simulink library "lib_rfsoc_fec"  (R2020b)
settings: Solver=VariableStepAuto  StartTime=0.0  StopTime=10.0  RelTol=1e-3
undefined symbols (not defined in the file): d, fs, generator_polynomial
libraries: commseqgen3 x84, hdlsllib x83, $bdroot x33, simulink x22, dspsigops x13
(part 3 of 4)

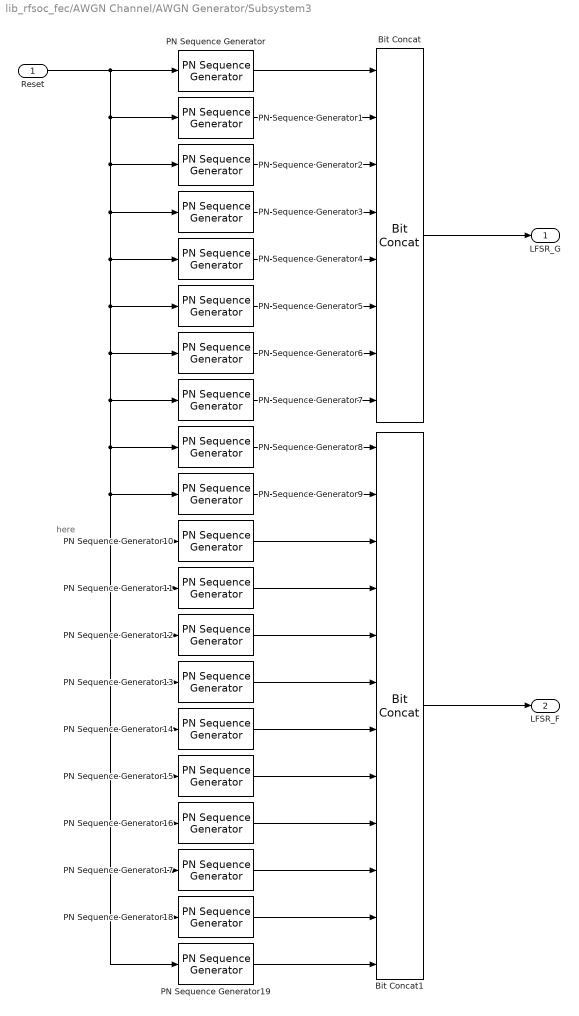
== system lib_rfsoc_fec/AWGN Channel/AWGN Generator/Subsystem3 ==
  note: here
  Reset : Inport
  Bit Concat : hdlsllib/Logic and Bit Operations/Bit Concat  numInputs=8
  Bit Concat1 : hdlsllib/Logic and Bit Operations/Bit Concat  numInputs=12
  PN Sequence Generator : commseqgen3/PN Sequence Generator  poly='z^13 + z^12 + z^11 + z^8 + 1'  ini_sta=[0 1 1 0 0 0 0 0 0 1 0 0 0]  outBitMaskSource=Dialog parameter  shift=0  outVarSiz=off  maxOutSizeMode=Dialog parameter  maxOutSize=[10 1]  Ts=-1  sampPerFrame=1  reset=on  bitPackedOutputs=off  outDataType=boolean  numPackedBits=8  bitPackDataSigned=off  bitPackedOutDType=Smallest integer
  PN Sequence Generator1 : commseqgen3/PN Sequence Generator  poly='z^13 + z^12 + z^11 + z^8 + 1'  ini_sta=[0 0 1 1 0 0 0 0 0 0 0 1 1]  outBitMaskSource=Dialog parameter  shift=0  outVarSiz=off  maxOutSizeMode=Dialog parameter  maxOutSize=[10 1]  Ts=-1  sampPerFrame=1  reset=on  bitPackedOutputs=off  outDataType=boolean  numPackedBits=8  bitPackDataSigned=off  bitPackedOutDType=Smallest integer
  PN Sequence Generator10 : commseqgen3/PN Sequence Generator  poly='z^13 + z^12 + z^11 + z^8 + 1'  ini_sta=[1 0 0 0 0 0 1 0 0 0 0 0 1]  outBitMaskSource=Dialog parameter  shift=0  outVarSiz=off  maxOutSizeMode=Dialog parameter  maxOutSize=[10 1]  Ts=-1  sampPerFrame=1  reset=on  bitPackedOutputs=off  outDataType=boolean  numPackedBits=8  bitPackDataSigned=off  bitPackedOutDType=Smallest integer
  PN Sequence Generator11 : commseqgen3/PN Sequence Generator  poly='z^13 + z^12 + z^11 + z^8 + 1'  ini_sta=[1 0 0 0 0 0 0 0 0 0 0 0 1]  outBitMaskSource=Dialog parameter  shift=0  outVarSiz=off  maxOutSizeMode=Dialog parameter  maxOutSize=[10 1]  Ts=-1  sampPerFrame=1  reset=on  bitPackedOutputs=off  outDataType=boolean  numPackedBits=8  bitPackDataSigned=off  bitPackedOutDType=Smallest integer
  PN Sequence Generator12 : commseqgen3/PN Sequence Generator  poly='z^13 + z^12 + z^11 + z^8 + 1'  ini_sta=[1 0 0 1 0 0 0 0 0 1 0 0 1]  outBitMaskSource=Dialog parameter  shift=0  outVarSiz=off  maxOutSizeMode=Dialog parameter  maxOutSize=[10 1]  Ts=-1  sampPerFrame=1  reset=on  bitPackedOutputs=off  outDataType=boolean  numPackedBits=8  bitPackDataSigned=off  bitPackedOutDType=Smallest integer
  PN Sequence Generator13 : commseqgen3/PN Sequence Generator  poly='z^13 + z^12 + z^11 + z^8 + 1'  ini_sta=[1 1 1 1 1 1 0 1 1 1 1 1 1]  outBitMaskSource=Dialog parameter  shift=0  outVarSiz=off  maxOutSizeMode=Dialog parameter  maxOutSize=[10 1]  Ts=-1  sampPerFrame=1  reset=on  bitPackedOutputs=off  outDataType=boolean  numPackedBits=8  bitPackDataSigned=off  bitPackedOutDType=Smallest integer
  PN Sequence Generator14 : commseqgen3/PN Sequence Generator  poly='z^13 + z^12 + z^11 + z^8 + 1'  ini_sta=[1 0 1 0 1 0 1 0 1 0 1 0 1]  outBitMaskSource=Dialog parameter  shift=0  outVarSiz=off  maxOutSizeMode=Dialog parameter  maxOutSize=[10 1]  Ts=-1  sampPerFrame=1  reset=on  bitPackedOutputs=off  outDataType=boolean  numPackedBits=8  bitPackDataSigned=off  bitPackedOutDType=Smallest integer
  PN Sequence Generator15 : commseqgen3/PN Sequence Generator  poly='z^13 + z^12 + z^11 + z^8 + 1'  ini_sta=[0 1 0 1 0 1 0 1 0 1 0 1 0]  outBitMaskSource=Dialog parameter  shift=0  outVarSiz=off  maxOutSizeMode=Dialog parameter  maxOutSize=[10 1]  Ts=-1  sampPerFrame=1  reset=on  bitPackedOutputs=off  outDataType=boolean  numPackedBits=8  bitPackDataSigned=off  bitPackedOutDType=Smallest integer
  PN Sequence Generator16 : commseqgen3/PN Sequence Generator  poly='z^13 + z^12 + z^11 + z^8 + 1'  ini_sta=[1 1 1 0 0 0 1 1 1 0 0 0 1]  outBitMaskSource=Dialog parameter  shift=0  outVarSiz=off  maxOutSizeMode=Dialog parameter  maxOutSize=[10 1]  Ts=-1  sampPerFrame=1  reset=on  bitPackedOutputs=off  outDataType=boolean  numPackedBits=8  bitPackDataSigned=off  bitPackedOutDType=Smallest integer
  PN Sequence Generator17 : commseqgen3/PN Sequence Generator  poly='z^13 + z^12 + z^11 + z^8 + 1'  ini_sta=[0 0 0 0 0 1 1 0 0 0 1 1 1]  outBitMaskSource=Dialog parameter  shift=0  outVarSiz=off  maxOutSizeMode=Dialog parameter  maxOutSize=[10 1]  Ts=-1  sampPerFrame=1  reset=on  bitPackedOutputs=off  outDataType=boolean  numPackedBits=8  bitPackDataSigned=off  bitPackedOutDType=Smallest integer
  PN Sequence Generator18 : commseqgen3/PN Sequence Generator  poly='z^13 + z^12 + z^11 + z^8 + 1'  ini_sta=[1 1 0 0 0 1 1 1 1 0 0 0 0]  outBitMaskSource=Dialog parameter  shift=0  outVarSiz=off  maxOutSizeMode=Dialog parameter  maxOutSize=[10 1]  Ts=-1  sampPerFrame=1  reset=on  bitPackedOutputs=off  outDataType=boolean  numPackedBits=8  bitPackDataSigned=off  bitPackedOutDType=Smallest integer
  PN Sequence Generator19 : commseqgen3/PN Sequence Generator  poly='z^13 + z^12 + z^11 + z^8 + 1'  ini_sta=[1 1 1 1 1 1 1 0 0 0 0 0 0]  outBitMaskSource=Dialog parameter  shift=0  outVarSiz=off  maxOutSizeMode=Dialog parameter  maxOutSize=[10 1]  Ts=-1  sampPerFrame=1  reset=on  bitPackedOutputs=off  outDataType=boolean  numPackedBits=8  bitPackDataSigned=off  bitPackedOutDType=Smallest integer
  PN Sequence Generator2 : commseqgen3/PN Sequence Generator  poly='z^13 + z^12 + z^11 + z^8 + 1'  ini_sta=[1 1 0 1 0 0 0 0 0 1 0 0 1]  outBitMaskSource=Dialog parameter  shift=0  outVarSiz=off  maxOutSizeMode=Dialog parameter  maxOutSize=[10 1]  Ts=-1  sampPerFrame=1  reset=on  bitPackedOutputs=off  outDataType=boolean  numPackedBits=8  bitPackDataSigned=off  bitPackedOutDType=Smallest integer
  PN Sequence Generator3 : commseqgen3/PN Sequence Generator  poly='z^13 + z^12 + z^11 + z^8 + 1'  ini_sta=[1 0 1 0 0 0 0 1 0 0 1 1 0]  outBitMaskSource=Dialog parameter  shift=0  outVarSiz=off  maxOutSizeMode=Dialog parameter  maxOutSize=[10 1]  Ts=-1  sampPerFrame=1  reset=on  bitPackedOutputs=off  outDataType=boolean  numPackedBits=8  bitPackDataSigned=off  bitPackedOutDType=Smallest integer
  PN Sequence Generator4 : commseqgen3/PN Sequence Generator  poly='z^13 + z^12 + z^11 + z^8 + 1'  ini_sta=[0 0 0 0 1 0 0 0 0 1 1 1 0]  outBitMaskSource=Dialog parameter  shift=0  outVarSiz=off  maxOutSizeMode=Dialog parameter  maxOutSize=[10 1]  Ts=-1  sampPerFrame=1  reset=on  bitPackedOutputs=off  outDataType=boolean  numPackedBits=8  bitPackDataSigned=off  bitPackedOutDType=Smallest integer
  PN Sequence Generator5 : commseqgen3/PN Sequence Generator  poly='z^13 + z^12 + z^11 + z^8 + 1'  ini_sta=[1 1 0 0 1 1 0 0 1 0 1 0 0]  outBitMaskSource=Dialog parameter  shift=0  outVarSiz=off  maxOutSizeMode=Dialog parameter  maxOutSize=[10 1]  Ts=-1  sampPerFrame=1  reset=on  bitPackedOutputs=off  outDataType=boolean  numPackedBits=8  bitPackDataSigned=off  bitPackedOutDType=Smallest integer
  PN Sequence Generator6 : commseqgen3/PN Sequence Generator  poly='z^13 + z^12 + z^11 + z^8 + 1'  ini_sta=[1 0 0 0 0 1 0 0 0 0 1 1 1]  outBitMaskSource=Dialog parameter  shift=0  outVarSiz=off  maxOutSizeMode=Dialog parameter  maxOutSize=[10 1]  Ts=-1  sampPerFrame=1  reset=on  bitPackedOutputs=off  outDataType=boolean  numPackedBits=8  bitPackDataSigned=off  bitPackedOutDType=Smallest integer
  PN Sequence Generator7 : commseqgen3/PN Sequence Generator  poly='z^13 + z^12 + z^11 + z^8 + 1'  ini_sta=[1 0 0 1 1 1 1 1 0 0 0 1 1]  outBitMaskSource=Dialog parameter  shift=0  outVarSiz=off  maxOutSizeMode=Dialog parameter  maxOutSize=[10 1]  Ts=-1  sampPerFrame=1  reset=on  bitPackedOutputs=off  outDataType=boolean  numPackedBits=8  bitPackDataSigned=off  bitPackedOutDType=Smallest integer
  PN Sequence Generator8 : commseqgen3/PN Sequence Generator  poly='z^13 + z^12 + z^11 + z^8 + 1'  ini_sta=[1 1 0 1 1 1 1 1 0 0 0 1 1]  outBitMaskSource=Dialog parameter  shift=0  outVarSiz=off  maxOutSizeMode=Dialog parameter  maxOutSize=[10 1]  Ts=-1  sampPerFrame=1  reset=on  bitPackedOutputs=off  outDataType=boolean  numPackedBits=8  bitPackDataSigned=off  bitPackedOutDType=Smallest integer
  PN Sequence Generator9 : commseqgen3/PN Sequence Generator  poly='z^13 + z^12 + z^11 + z^8 + 1'  ini_sta=[0 1 0 1 1 0 0 1 0 0 0 1 1]  outBitMaskSource=Dialog parameter  shift=0  outVarSiz=off  maxOutSizeMode=Dialog parameter  maxOutSize=[10 1]  Ts=-1  sampPerFrame=1  reset=on  bitPackedOutputs=off  outDataType=boolean  numPackedBits=8  bitPackDataSigned=off  bitPackedOutDType=Smallest integer
  LFSR_G : Outport
  LFSR_F : Outport  Port=2
  wires:
  PN Sequence Generator11/1 -> Bit Concat1/4
  PN Sequence Generator10/1 -> Bit Concat1/3
  PN Sequence Generator9/1 -> Bit Concat1/2
  PN Sequence Generator8/1 -> Bit Concat1/1
  Bit Concat1/1 -> LFSR_F/1
  Bit Concat/1 -> LFSR_G/1
  Reset/1 -> PN Sequence Generator/1, PN Sequence Generator2/1, PN Sequence Generator3/1, PN Sequence Generator8/1, PN Sequence Generator9/1, PN Sequence Generator11/1, PN Sequence Generator18/1, PN Sequence Generator19/1, PN Sequence Generator17/1, PN Sequence Generator16/1, PN Sequence Generator15/1, PN Sequence Generator14/1, PN Sequence Generator13/1, PN Sequence Generator12/1, PN Sequence Generator10/1, PN Sequence Generator7/1, PN Sequence Generator6/1, PN Sequence Generator5/1, PN Sequence Generator4/1, PN Sequence Generator1/1
  PN Sequence Generator18/1 -> Bit Concat1/11
  PN Sequence Generator13/1 -> Bit Concat1/6
  PN Sequence Generator14/1 -> Bit Concat1/7
  PN Sequence Generator12/1 -> Bit Concat1/5
  PN Sequence Generator15/1 -> Bit Concat1/8
  PN Sequence Generator16/1 -> Bit Concat1/9
  PN Sequence Generator17/1 -> Bit Concat1/10
  PN Sequence Generator19/1 -> Bit Concat1/12
  PN Sequence Generator7/1 -> Bit Concat/8
  PN Sequence Generator6/1 -> Bit Concat/7
  PN Sequence Generator5/1 -> Bit Concat/6
  PN Sequence Generator2/1 -> Bit Concat/3
  PN Sequence Generator1/1 -> Bit Concat/2
  PN Sequence Generator4/1 -> Bit Concat/5
  PN Sequence Generator3/1 -> Bit Concat/4
  PN Sequence Generator/1 -> Bit Concat/1

== system lib_rfsoc_fec/AWGN Channel/sample_and_hold/tvalid hold ==
  In1 : Inport
  Compare To Constant : simulink/Logic and Bit Operations/Compare To Constant  relop===  const=7  OutDataTypeStr=boolean
  Delay1 : Delay  DelayLength=1
  HDL Counter : hdlsllib/Sources/HDL Counter  CountType=Count limited  CountInit=0  CountStep=1  CountMax=7  CountFromType=Initial value  CountFrom=0  CountResetPort=off  CountLoadPort=off  CountEnbPort=on  CountDirPort=off  CountDataType=Unsigned  CountWordLen=3  CountFracLen=0  CountSampTime=1
  OR : Logic  Operator=OR  IconShape=distinctive  AllPortsSameDT=off  OutDataTypeStr=boolean
  Sample and Hold1 : dspsigops/Sample and Hold  trig=Rising edge  initCond=0  latchinput=off
  " " : Outport
  wires:
  HDL Counter/1 -> Compare To Constant/1
  Delay1/1 -> OR/1
  OR/1 -> Sample and Hold1/Trigger
  Compare To Constant/1 -> Delay1/1
  Sample and Hold1/1 -> " "/1, HDL Counter/1
  In1/1 -> Sample and Hold1/1, OR/2

== system lib_rfsoc_fec/QAM Mapping/Buffer/sample_and_hold ==
  s_axis_tvalid : Inport
  s_axis_tdata : Inport  Port=2
  Sample and Hold : dspsigops/Sample and Hold  trig=Rising edge  initCond=0  latchinput=off
  tvalid hold : Subsystem
  " valid_out" : Outport
  " m_axis_tdata" : Outport  Port=2
  wires:
  s_axis_tvalid/1 -> Sample and Hold/Trigger, tvalid hold/1(In1)
  tvalid hold/1(" ") -> " valid_out"/1
  s_axis_tdata/1 -> Sample and Hold/1
  Sample and Hold/1 -> " m_axis_tdata"/1

== system lib_rfsoc_fec/QAM Mapping/Buffer/sample_and_hold1 ==
  s_axis_tvalid : Inport
  s_axis_tdata : Inport  Port=2
  Sample and Hold : dspsigops/Sample and Hold  trig=Rising edge  initCond=0  latchinput=off
  tvalid hold : Subsystem
  " valid_out" : Outport
  " m_axis_tdata" : Outport  Port=2
  wires:
  Sample and Hold/1 -> " m_axis_tdata"/1
  s_axis_tdata/1 -> Sample and Hold/1
  tvalid hold/1(" ") -> " valid_out"/1
  s_axis_tvalid/1 -> tvalid hold/1(In1), Sample and Hold/Trigger

== system lib_rfsoc_fec/QAM Mapping/Buffer/sample_and_hold2 ==
  s_axis_tvalid : Inport
  s_axis_tdata : Inport  Port=2
  Sample and Hold : dspsigops/Sample and Hold  trig=Rising edge  initCond=0  latchinput=off
  tvalid hold : Subsystem
  " valid_out" : Outport
  " m_axis_tdata" : Outport  Port=2
  wires:
  s_axis_tvalid/1 -> Sample and Hold/Trigger, tvalid hold/1(In1)
  tvalid hold/1(" ") -> " valid_out"/1
  s_axis_tdata/1 -> Sample and Hold/1
  Sample and Hold/1 -> " m_axis_tdata"/1

== system lib_rfsoc_fec/QAM Mapping/Buffer/sample_and_hold3 ==
  s_axis_tvalid : Inport
  s_axis_tdata : Inport  Port=2
  Sample and Hold : dspsigops/Sample and Hold  trig=Rising edge  initCond=0  latchinput=off
  tvalid hold : Subsystem
  " valid_out" : Outport
  " m_axis_tdata" : Outport  Port=2
  wires:
  Sample and Hold/1 -> " m_axis_tdata"/1
  s_axis_tdata/1 -> Sample and Hold/1
  tvalid hold/1(" ") -> " valid_out"/1
  s_axis_tvalid/1 -> tvalid hold/1(In1), Sample and Hold/Trigger

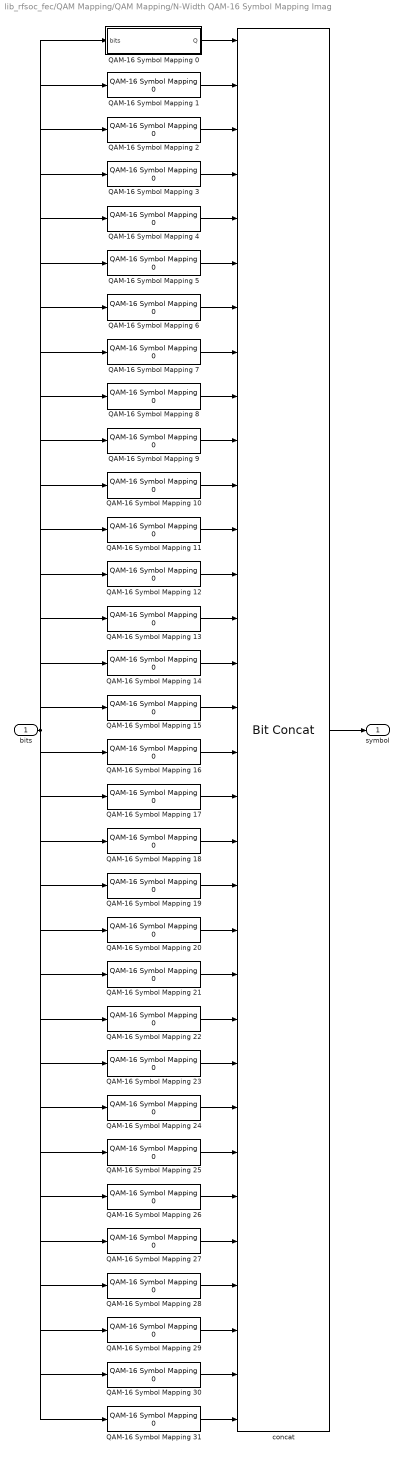
== system lib_rfsoc_fec/QAM Mapping/QAM Mapping/N-Width QAM-16 Symbol Mapping Imag ==
  bits : Inport
  QAM-16 Symbol Mapping 0 : Subsystem  mask{n=124}
  QAM-16 Symbol Mapping 1 : $bdroot/QAM Mapping/QAM Mapping/N-Width QAM-16 Symbol Mapping Imag/QAM-16 Symbol Mapping 0  n=120
  QAM-16 Symbol Mapping 10 : $bdroot/QAM Mapping/QAM Mapping/N-Width QAM-16 Symbol Mapping Imag/QAM-16 Symbol Mapping 0  n=84
  QAM-16 Symbol Mapping 11 : $bdroot/QAM Mapping/QAM Mapping/N-Width QAM-16 Symbol Mapping Imag/QAM-16 Symbol Mapping 0  n=80
  QAM-16 Symbol Mapping 12 : $bdroot/QAM Mapping/QAM Mapping/N-Width QAM-16 Symbol Mapping Imag/QAM-16 Symbol Mapping 0  n=76
  QAM-16 Symbol Mapping 13 : $bdroot/QAM Mapping/QAM Mapping/N-Width QAM-16 Symbol Mapping Imag/QAM-16 Symbol Mapping 0  n=72
  QAM-16 Symbol Mapping 14 : $bdroot/QAM Mapping/QAM Mapping/N-Width QAM-16 Symbol Mapping Imag/QAM-16 Symbol Mapping 0  n=68
  QAM-16 Symbol Mapping 15 : $bdroot/QAM Mapping/QAM Mapping/N-Width QAM-16 Symbol Mapping Imag/QAM-16 Symbol Mapping 0  n=64
  QAM-16 Symbol Mapping 16 : $bdroot/QAM Mapping/QAM Mapping/N-Width QAM-16 Symbol Mapping Imag/QAM-16 Symbol Mapping 0  n=60
  QAM-16 Symbol Mapping 17 : $bdroot/QAM Mapping/QAM Mapping/N-Width QAM-16 Symbol Mapping Imag/QAM-16 Symbol Mapping 0  n=56
  QAM-16 Symbol Mapping 18 : $bdroot/QAM Mapping/QAM Mapping/N-Width QAM-16 Symbol Mapping Imag/QAM-16 Symbol Mapping 0  n=52
  QAM-16 Symbol Mapping 19 : $bdroot/QAM Mapping/QAM Mapping/N-Width QAM-16 Symbol Mapping Imag/QAM-16 Symbol Mapping 0  n=48
  QAM-16 Symbol Mapping 2 : $bdroot/QAM Mapping/QAM Mapping/N-Width QAM-16 Symbol Mapping Imag/QAM-16 Symbol Mapping 0  n=116
  QAM-16 Symbol Mapping 20 : $bdroot/QAM Mapping/QAM Mapping/N-Width QAM-16 Symbol Mapping Imag/QAM-16 Symbol Mapping 0  n=44
  QAM-16 Symbol Mapping 21 : $bdroot/QAM Mapping/QAM Mapping/N-Width QAM-16 Symbol Mapping Imag/QAM-16 Symbol Mapping 0  n=40
  QAM-16 Symbol Mapping 22 : $bdroot/QAM Mapping/QAM Mapping/N-Width QAM-16 Symbol Mapping Imag/QAM-16 Symbol Mapping 0  n=36
  QAM-16 Symbol Mapping 23 : $bdroot/QAM Mapping/QAM Mapping/N-Width QAM-16 Symbol Mapping Imag/QAM-16 Symbol Mapping 0  n=32
  QAM-16 Symbol Mapping 24 : $bdroot/QAM Mapping/QAM Mapping/N-Width QAM-16 Symbol Mapping Imag/QAM-16 Symbol Mapping 0  n=28
  QAM-16 Symbol Mapping 25 : $bdroot/QAM Mapping/QAM Mapping/N-Width QAM-16 Symbol Mapping Imag/QAM-16 Symbol Mapping 0  n=24
  QAM-16 Symbol Mapping 26 : $bdroot/QAM Mapping/QAM Mapping/N-Width QAM-16 Symbol Mapping Imag/QAM-16 Symbol Mapping 0  n=20
  QAM-16 Symbol Mapping 27 : $bdroot/QAM Mapping/QAM Mapping/N-Width QAM-16 Symbol Mapping Imag/QAM-16 Symbol Mapping 0  n=16
  QAM-16 Symbol Mapping 28 : $bdroot/QAM Mapping/QAM Mapping/N-Width QAM-16 Symbol Mapping Imag/QAM-16 Symbol Mapping 0  n=12
  QAM-16 Symbol Mapping 29 : $bdroot/QAM Mapping/QAM Mapping/N-Width QAM-16 Symbol Mapping Imag/QAM-16 Symbol Mapping 0  n=8
  QAM-16 Symbol Mapping 3 : $bdroot/QAM Mapping/QAM Mapping/N-Width QAM-16 Symbol Mapping Imag/QAM-16 Symbol Mapping 0  n=112
  QAM-16 Symbol Mapping 30 : $bdroot/QAM Mapping/QAM Mapping/N-Width QAM-16 Symbol Mapping Imag/QAM-16 Symbol Mapping 0  n=4
  QAM-16 Symbol Mapping 31 : $bdroot/QAM Mapping/QAM Mapping/N-Width QAM-16 Symbol Mapping Imag/QAM-16 Symbol Mapping 0  n=0
  QAM-16 Symbol Mapping 4 : $bdroot/QAM Mapping/QAM Mapping/N-Width QAM-16 Symbol Mapping Imag/QAM-16 Symbol Mapping 0  n=108
  QAM-16 Symbol Mapping 5 : $bdroot/QAM Mapping/QAM Mapping/N-Width QAM-16 Symbol Mapping Imag/QAM-16 Symbol Mapping 0  n=104
  QAM-16 Symbol Mapping 6 : $bdroot/QAM Mapping/QAM Mapping/N-Width QAM-16 Symbol Mapping Imag/QAM-16 Symbol Mapping 0  n=100
  QAM-16 Symbol Mapping 7 : $bdroot/QAM Mapping/QAM Mapping/N-Width QAM-16 Symbol Mapping Imag/QAM-16 Symbol Mapping 0  n=96
  QAM-16 Symbol Mapping 8 : $bdroot/QAM Mapping/QAM Mapping/N-Width QAM-16 Symbol Mapping Imag/QAM-16 Symbol Mapping 0  n=92
  QAM-16 Symbol Mapping 9 : $bdroot/QAM Mapping/QAM Mapping/N-Width QAM-16 Symbol Mapping Imag/QAM-16 Symbol Mapping 0  n=88
  concat : hdlsllib/Logic and Bit Operations/Bit Concat  numInputs=32
  symbol : Outport
  wires:
  bits/1 -> QAM-16 Symbol Mapping 0/1(bits), QAM-16 Symbol Mapping 1/1, QAM-16 Symbol Mapping 2/1, QAM-16 Symbol Mapping 3/1, QAM-16 Symbol Mapping 4/1, QAM-16 Symbol Mapping 5/1, QAM-16 Symbol Mapping 6/1, QAM-16 Symbol Mapping 7/1, QAM-16 Symbol Mapping 8/1, QAM-16 Symbol Mapping 9/1, QAM-16 Symbol Mapping 10/1, QAM-16 Symbol Mapping 11/1, QAM-16 Symbol Mapping 12/1, QAM-16 Symbol Mapping 13/1, QAM-16 Symbol Mapping 14/1, QAM-16 Symbol Mapping 15/1, QAM-16 Symbol Mapping 16/1, QAM-16 Symbol Mapping 17/1, QAM-16 Symbol Mapping 18/1, QAM-16 Symbol Mapping 19/1, QAM-16 Symbol Mapping 20/1, QAM-16 Symbol Mapping 21/1, QAM-16 Symbol Mapping 22/1, QAM-16 Symbol Mapping 23/1, QAM-16 Symbol Mapping 24/1, QAM-16 Symbol Mapping 25/1, QAM-16 Symbol Mapping 26/1, QAM-16 Symbol Mapping 27/1, QAM-16 Symbol Mapping 28/1, QAM-16 Symbol Mapping 29/1, QAM-16 Symbol Mapping 30/1, QAM-16 Symbol Mapping 31/1
  QAM-16 Symbol Mapping 0/1(Q) -> concat/1
  QAM-16 Symbol Mapping 1/1 -> concat/2
  QAM-16 Symbol Mapping 2/1 -> concat/3
  QAM-16 Symbol Mapping 3/1 -> concat/4
  QAM-16 Symbol Mapping 4/1 -> concat/5
  QAM-16 Symbol Mapping 5/1 -> concat/6
  QAM-16 Symbol Mapping 6/1 -> concat/7
  QAM-16 Symbol Mapping 7/1 -> concat/8
  QAM-16 Symbol Mapping 8/1 -> concat/9
  QAM-16 Symbol Mapping 9/1 -> concat/10
  QAM-16 Symbol Mapping 10/1 -> concat/11
  QAM-16 Symbol Mapping 11/1 -> concat/12
  QAM-16 Symbol Mapping 12/1 -> concat/13
  QAM-16 Symbol Mapping 13/1 -> concat/14
  QAM-16 Symbol Mapping 14/1 -> concat/15
  QAM-16 Symbol Mapping 15/1 -> concat/16
  QAM-16 Symbol Mapping 16/1 -> concat/17
  QAM-16 Symbol Mapping 17/1 -> concat/18
  QAM-16 Symbol Mapping 18/1 -> concat/19
  QAM-16 Symbol Mapping 19/1 -> concat/20
  QAM-16 Symbol Mapping 20/1 -> concat/21
  QAM-16 Symbol Mapping 21/1 -> concat/22
  QAM-16 Symbol Mapping 22/1 -> concat/23
  QAM-16 Symbol Mapping 23/1 -> concat/24
  QAM-16 Symbol Mapping 24/1 -> concat/25
  QAM-16 Symbol Mapping 25/1 -> concat/26
  QAM-16 Symbol Mapping 26/1 -> concat/27
  QAM-16 Symbol Mapping 27/1 -> concat/28
  QAM-16 Symbol Mapping 28/1 -> concat/29
  QAM-16 Symbol Mapping 29/1 -> concat/30
  QAM-16 Symbol Mapping 30/1 -> concat/31
  QAM-16 Symbol Mapping 31/1 -> concat/32
  concat/1 -> symbol/1

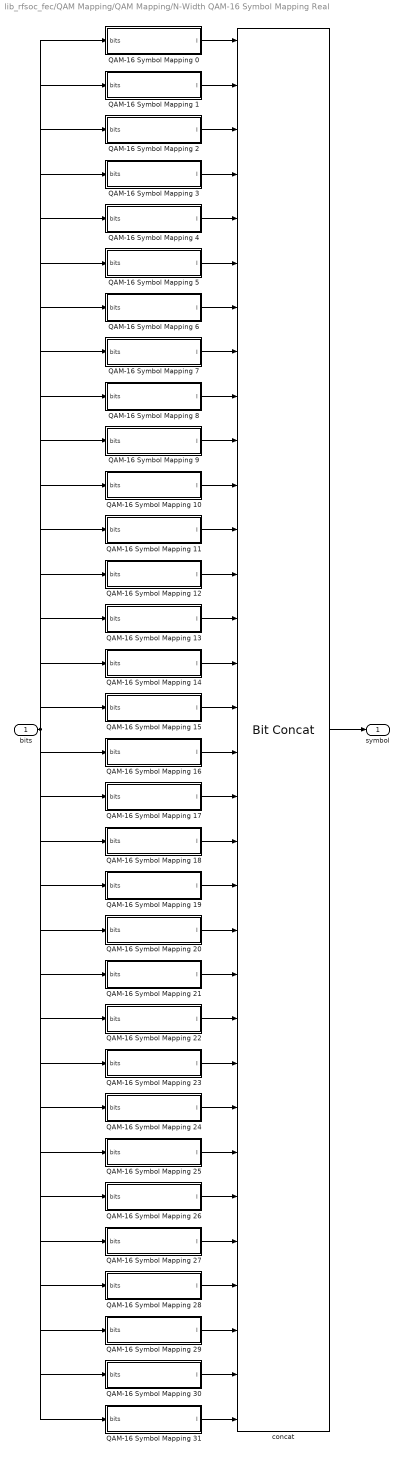
== system lib_rfsoc_fec/QAM Mapping/QAM Mapping/N-Width QAM-16 Symbol Mapping Real ==
  bits : Inport
  QAM-16 Symbol Mapping 0 : Subsystem  mask{n=124}
  QAM-16 Symbol Mapping 1 : Subsystem  mask{n=120}
  QAM-16 Symbol Mapping 10 : Subsystem  mask{n=84}
  QAM-16 Symbol Mapping 11 : Subsystem  mask{n=80}
  QAM-16 Symbol Mapping 12 : Subsystem  mask{n=76}
  QAM-16 Symbol Mapping 13 : Subsystem  mask{n=72}
  QAM-16 Symbol Mapping 14 : Subsystem  mask{n=68}
  QAM-16 Symbol Mapping 15 : Subsystem  mask{n=64}
  QAM-16 Symbol Mapping 16 : Subsystem  mask{n=60}
  QAM-16 Symbol Mapping 17 : Subsystem  mask{n=56}
  QAM-16 Symbol Mapping 18 : Subsystem  mask{n=52}
  QAM-16 Symbol Mapping 19 : Subsystem  mask{n=48}
  QAM-16 Symbol Mapping 2 : Subsystem  mask{n=116}
  QAM-16 Symbol Mapping 20 : Subsystem  mask{n=44}
  QAM-16 Symbol Mapping 21 : Subsystem  mask{n=40}
  QAM-16 Symbol Mapping 22 : Subsystem  mask{n=36}
  QAM-16 Symbol Mapping 23 : Subsystem  mask{n=32}
  QAM-16 Symbol Mapping 24 : Subsystem  mask{n=28}
  QAM-16 Symbol Mapping 25 : Subsystem  mask{n=24}
  QAM-16 Symbol Mapping 26 : Subsystem  mask{n=20}
  QAM-16 Symbol Mapping 27 : Subsystem  mask{n=16}
  QAM-16 Symbol Mapping 28 : Subsystem  mask{n=12}
  QAM-16 Symbol Mapping 29 : Subsystem  mask{n=8}
  QAM-16 Symbol Mapping 3 : Subsystem  mask{n=112}
  QAM-16 Symbol Mapping 30 : Subsystem  mask{n=4}
  QAM-16 Symbol Mapping 31 : Subsystem  mask{n=0}
  QAM-16 Symbol Mapping 4 : Subsystem  mask{n=108}
  QAM-16 Symbol Mapping 5 : Subsystem  mask{n=104}
  QAM-16 Symbol Mapping 6 : Subsystem  mask{n=100}
  QAM-16 Symbol Mapping 7 : Subsystem  mask{n=96}
  QAM-16 Symbol Mapping 8 : Subsystem  mask{n=92}
  QAM-16 Symbol Mapping 9 : Subsystem  mask{n=88}
  concat : hdlsllib/Logic and Bit Operations/Bit Concat  numInputs=32
  symbol : Outport
  wires:
  concat/1 -> symbol/1
  QAM-16 Symbol Mapping 31/1(I) -> concat/32
  QAM-16 Symbol Mapping 30/1(I) -> concat/31
  QAM-16 Symbol Mapping 29/1(I) -> concat/30
  QAM-16 Symbol Mapping 28/1(I) -> concat/29
  QAM-16 Symbol Mapping 27/1(I) -> concat/28
  QAM-16 Symbol Mapping 26/1(I) -> concat/27
  QAM-16 Symbol Mapping 25/1(I) -> concat/26
  QAM-16 Symbol Mapping 24/1(I) -> concat/25
  QAM-16 Symbol Mapping 23/1(I) -> concat/24
  QAM-16 Symbol Mapping 22/1(I) -> concat/23
  QAM-16 Symbol Mapping 21/1(I) -> concat/22
  QAM-16 Symbol Mapping 20/1(I) -> concat/21
  QAM-16 Symbol Mapping 19/1(I) -> concat/20
  QAM-16 Symbol Mapping 18/1(I) -> concat/19
  QAM-16 Symbol Mapping 17/1(I) -> concat/18
  QAM-16 Symbol Mapping 16/1(I) -> concat/17
  QAM-16 Symbol Mapping 15/1(I) -> concat/16
  QAM-16 Symbol Mapping 14/1(I) -> concat/15
  QAM-16 Symbol Mapping 13/1(I) -> concat/14
  QAM-16 Symbol Mapping 12/1(I) -> concat/13
  QAM-16 Symbol Mapping 11/1(I) -> concat/12
  QAM-16 Symbol Mapping 10/1(I) -> concat/11
  QAM-16 Symbol Mapping 9/1(I) -> concat/10
  QAM-16 Symbol Mapping 8/1(I) -> concat/9
  QAM-16 Symbol Mapping 7/1(I) -> concat/8
  QAM-16 Symbol Mapping 6/1(I) -> concat/7
  QAM-16 Symbol Mapping 5/1(I) -> concat/6
  QAM-16 Symbol Mapping 4/1(I) -> concat/5
  QAM-16 Symbol Mapping 3/1(I) -> concat/4
  QAM-16 Symbol Mapping 2/1(I) -> concat/3
  QAM-16 Symbol Mapping 1/1(I) -> concat/2
  QAM-16 Symbol Mapping 0/1(I) -> concat/1
  bits/1 -> QAM-16 Symbol Mapping 31/1(bits), QAM-16 Symbol Mapping 30/1(bits), QAM-16 Symbol Mapping 29/1(bits), QAM-16 Symbol Mapping 28/1(bits), QAM-16 Symbol Mapping 27/1(bits), QAM-16 Symbol Mapping 26/1(bits), QAM-16 Symbol Mapping 25/1(bits), QAM-16 Symbol Mapping 24/1(bits), QAM-16 Symbol Mapping 23/1(bits), QAM-16 Symbol Mapping 22/1(bits), QAM-16 Symbol Mapping 21/1(bits), QAM-16 Symbol Mapping 20/1(bits), QAM-16 Symbol Mapping 19/1(bits), QAM-16 Symbol Mapping 18/1(bits), QAM-16 Symbol Mapping 17/1(bits), QAM-16 Symbol Mapping 16/1(bits), QAM-16 Symbol Mapping 15/1(bits), QAM-16 Symbol Mapping 14/1(bits), QAM-16 Symbol Mapping 13/1(bits), QAM-16 Symbol Mapping 12/1(bits), QAM-16 Symbol Mapping 11/1(bits), QAM-16 Symbol Mapping 10/1(bits), QAM-16 Symbol Mapping 9/1(bits), QAM-16 Symbol Mapping 8/1(bits), QAM-16 Symbol Mapping 7/1(bits), QAM-16 Symbol Mapping 6/1(bits), QAM-16 Symbol Mapping 5/1(bits), QAM-16 Symbol Mapping 4/1(bits), QAM-16 Symbol Mapping 3/1(bits), QAM-16 Symbol Mapping 2/1(bits), QAM-16 Symbol Mapping 1/1(bits), QAM-16 Symbol Mapping 0/1(bits)

== system lib_rfsoc_fec/Random Number Generator/byte_count/falling_edge ==
  in : Inport
  Data Type Conversion1 : DataTypeConversion  OutDataTypeStr=boolean  SaturateOnIntegerOverflow=on  RndMeth=Zero
  Delay15 : Delay  DelayLength=1  InitialCondition=1  InputProcessing=Columns as channels (frame based)
  Logical Operator1 : Logic  Operator=NOT  Inputs=1
  Logical Operator3 : Logic
  pulse : Outport
  wires:
  Logical Operator3/1 -> pulse/1
  in/1 -> Data Type Conversion1/1
  Delay15/1 -> Logical Operator3/2
  Data Type Conversion1/1 -> Logical Operator1/1, Delay15/1
  Logical Operator1/1 -> Logical Operator3/1

== system lib_rfsoc_fec/Random Number Generator/concat/mask_generator ==
  diff : Inport
  sel : Inport  Port=2
  1-D Lookup Table{,1..3} (4 alike) : Lookup_n-D  NumberOfTableDimensions=1  BreakpointsForDimension1=[0:32]  Table=[ 0 2.^[1:32] - 1]  ExtrapMethod=Clip  InternalRulePriority=Speed  OutDataTypeStr=fixdt(0,32,0)  RndMeth=Simplest  InputSameDT=on
  Bit Concat1 : hdlsllib/Logic and Bit Operations/Bit Concat  numInputs=4
  Constant : Constant  Value=96  OutDataTypeStr=uint8  SampleTime=-1
  Constant1 : Constant  Value=2^128 - 1  OutDataTypeStr=fixdt(0,128,0)  SampleTime=-1
  Constant6 : Constant  Value=128  OutDataTypeStr=uint8  SampleTime=-1
  Constant7 : Constant  Value=64  OutDataTypeStr=uint8  SampleTime=-1
  Constant8 : Constant  Value=32  OutDataTypeStr=uint8  SampleTime=-1
  Multiport Switch : MultiPortSwitch  DataPortOrder=Zero-based contiguous  Inputs=2  zeroidx=on
  Saturation{,1..3} (4 alike) : Saturate  UpperLimit=32  LowerLimit=0
  Subtract : Sum  Inputs=+-  SaturateOnIntegerOverflow=on
  Subtract1 : Sum  Inputs=+-  SaturateOnIntegerOverflow=on
  Subtract2 : Sum  Inputs=+-  SaturateOnIntegerOverflow=on
  Subtract3 : Sum  Inputs=+-  OutDataTypeStr=uint8
  falling_edge : Subsystem
  mask : Outport
  wires:
  falling_edge/1(pulse) -> Multiport Switch/1
  sel/1 -> falling_edge/1(in)
  1-D Lookup Table1/1 -> Bit Concat1/2
  1-D Lookup Table/1 -> Bit Concat1/1
  1-D Lookup Table3/1 -> Bit Concat1/4
  Constant/1 -> Subtract/2
  Subtract/1 -> Saturation/1
  diff/1 -> Subtract3/2
  Subtract2/1 -> Saturation2/1
  Subtract1/1 -> Saturation1/1
  Constant7/1 -> Subtract1/2
  Saturation/1 -> 1-D Lookup Table/1
  1-D Lookup Table2/1 -> Bit Concat1/3
  Saturation1/1 -> 1-D Lookup Table1/1
  Saturation2/1 -> 1-D Lookup Table2/1
  Saturation3/1 -> 1-D Lookup Table3/1
  Constant8/1 -> Subtract2/2
  Bit Concat1/1 -> Multiport Switch/3
  Subtract3/1 -> Saturation3/1, Subtract2/1, Subtract1/1, Subtract/1
  Constant6/1 -> Subtract3/1
  Constant1/1 -> Multiport Switch/2
  Multiport Switch/1 -> mask/1

== system lib_rfsoc_fec/Random Number Generator/interface_creator/latch1 ==
  data_in : Inport
  en : Inport  Port=2
  Delay16 : Delay  DelayLength=1
  Multiport Switch : MultiPortSwitch  DataPortOrder=Zero-based contiguous  Inputs=2  zeroidx=on
  data_out : Outport
  wires:
  Multiport Switch/1 -> data_out/1, Delay16/1
  Delay16/1 -> Multiport Switch/2
  en/1 -> Multiport Switch/1
  data_in/1 -> Multiport Switch/3

== system lib_rfsoc_fec/Random Number Generator/interface_creator/latch10 ==
  data_in : Inport
  en : Inport  Port=2
  Delay16 : Delay  DelayLength=1
  Multiport Switch : MultiPortSwitch  DataPortOrder=Zero-based contiguous  Inputs=2  zeroidx=on
  data_out : Outport
  wires:
  en/1 -> Multiport Switch/1
  data_in/1 -> Multiport Switch/3
  Delay16/1 -> Multiport Switch/2
  Multiport Switch/1 -> Delay16/1, data_out/1

== system lib_rfsoc_fec/Random Number Generator/interface_creator/latch2 ==
  data_in : Inport
  en : Inport  Port=2
  Delay16 : Delay  DelayLength=1
  Multiport Switch : MultiPortSwitch  DataPortOrder=Zero-based contiguous  Inputs=2  zeroidx=on
  data_out : Outport
  wires:
  data_in/1 -> Multiport Switch/3
  en/1 -> Multiport Switch/1
  Delay16/1 -> Multiport Switch/2
  Multiport Switch/1 -> Delay16/1, data_out/1

== system lib_rfsoc_fec/Random Number Generator/interface_creator/latch4 ==
  data : Inport
  reset : Inport  Port=2
  Delay16 : Delay  DelayLength=1
  Multiport Switch : MultiPortSwitch  DataPortOrder=Zero-based contiguous  Inputs=2  zeroidx=on
  OR1 : Logic  Operator=OR  IconShape=distinctive  AllPortsSameDT=off  OutDataTypeStr=boolean
  data_out : Outport
  wires:
  Multiport Switch/1 -> data_out/1, Delay16/1
  Delay16/1 -> Multiport Switch/2
  OR1/1 -> Multiport Switch/1
  reset/1 -> OR1/1
  data/1 -> OR1/2, Multiport Switch/3

== system lib_rfsoc_fec/Random Number Generator/interface_creator/latch5 ==
  data : Inport
  reset : Inport  Port=2
  Delay16 : Delay  DelayLength=1
  Multiport Switch : MultiPortSwitch  DataPortOrder=Zero-based contiguous  Inputs=2  zeroidx=on
  OR1 : Logic  Operator=OR  IconShape=distinctive  AllPortsSameDT=off  OutDataTypeStr=boolean
  data_out : Outport
  wires:
  data/1 -> Multiport Switch/3, OR1/2
  reset/1 -> OR1/1
  OR1/1 -> Multiport Switch/1
  Delay16/1 -> Multiport Switch/2
  Multiport Switch/1 -> Delay16/1, data_out/1

== system lib_rfsoc_fec/Random Number Generator/interface_creator/latch6 ==
  data : Inport
  reset : Inport  Port=2
  Delay16 : Delay  DelayLength=1
  Multiport Switch : MultiPortSwitch  DataPortOrder=Zero-based contiguous  Inputs=2  zeroidx=on
  OR1 : Logic  Operator=OR  IconShape=distinctive  AllPortsSameDT=off  OutDataTypeStr=boolean
  data_out : Outport
  wires:
  Multiport Switch/1 -> data_out/1, Delay16/1
  Delay16/1 -> Multiport Switch/2
  OR1/1 -> Multiport Switch/1
  reset/1 -> OR1/1
  data/1 -> OR1/2, Multiport Switch/3

== system lib_rfsoc_fec/Random Number Generator/interface_creator/latch7 ==
  data_in : Inport
  en : Inport  Port=2
  Delay16 : Delay  DelayLength=1
  Multiport Switch : MultiPortSwitch  DataPortOrder=Zero-based contiguous  Inputs=2  zeroidx=on
  data_out : Outport
  wires:
  en/1 -> Multiport Switch/1
  Multiport Switch/1 -> data_out/1, Delay16/1
  Delay16/1 -> Multiport Switch/2
  data_in/1 -> Multiport Switch/3

== system lib_rfsoc_fec/Random Number Generator/interface_creator/latch8 ==
  data_in : Inport
  en : Inport  Port=2
  Delay16 : Delay  DelayLength=1
  Multiport Switch : MultiPortSwitch  DataPortOrder=Zero-based contiguous  Inputs=2  zeroidx=on
  data_out : Outport
  wires:
  en/1 -> Multiport Switch/1
  data_in/1 -> Multiport Switch/3
  Delay16/1 -> Multiport Switch/2
  Multiport Switch/1 -> Delay16/1, data_out/1

== system lib_rfsoc_fec/Random Number Generator/interface_creator/latch9 ==
  data_in : Inport
  en : Inport  Port=2
  Delay16 : Delay  DelayLength=1
  Multiport Switch : MultiPortSwitch  DataPortOrder=Zero-based contiguous  Inputs=2  zeroidx=on
  data_out : Outport
  wires:
  Multiport Switch/1 -> data_out/1, Delay16/1
  Delay16/1 -> Multiport Switch/2
  data_in/1 -> Multiport Switch/3
  en/1 -> Multiport Switch/1

== system lib_rfsoc_fec/Random Number Generator/interface_creator/rising_edge ==
  in : Inport
  Data Type Conversion1 : DataTypeConversion  OutDataTypeStr=boolean  SaturateOnIntegerOverflow=on  RndMeth=Zero
  Delay15 : Delay  DelayLength=1  InitialCondition=1  InputProcessing=Columns as channels (frame based)
  Logical Operator2 : Logic  Operator=NOT  Inputs=1
  Logical Operator3 : Logic
  pulse : Outport
  wires:
  Logical Operator2/1 -> Logical Operator3/2
  in/1 -> Data Type Conversion1/1
  Data Type Conversion1/1 -> Logical Operator3/1, Delay15/1
  Logical Operator3/1 -> pulse/1
  Delay15/1 -> Logical Operator2/1

== system lib_rfsoc_fec/Soft Demodulation/Soft Demodulation/Subsystem ==
  enb : Inport
  1-D Lookup Table : Lookup_n-D  NumberOfTableDimensions=1  BreakpointsForDimension1=[0:3]  IndexSearchMethod=Evenly spaced points  Table=[3 3 3 -1]  InterpMethod=Flat  DiagnosticForOutOfRangeInput=Error  InternalRulePriority=Speed  OutDataTypeStr=fixdt(1,3,0)  RndMeth=Simplest  InputSameDT=on
  1-D Lookup Table1 : Lookup_n-D  NumberOfTableDimensions=1  BreakpointsForDimension1=[0:3]  IndexSearchMethod=Evenly spaced points  Table=[1 1 3 -1]  InterpMethod=Flat  DiagnosticForOutOfRangeInput=Error  InternalRulePriority=Speed  OutDataTypeStr=fixdt(1,3,0)  RndMeth=Simplest  InputSameDT=on
  1-D Lookup Table2 : Lookup_n-D  NumberOfTableDimensions=1  BreakpointsForDimension1=[0:3]  IndexSearchMethod=Evenly spaced points  Table=[-1 -1 3 -1]  InterpMethod=Flat  DiagnosticForOutOfRangeInput=Error  InternalRulePriority=Speed  OutDataTypeStr=fixdt(1,3,0)  RndMeth=Simplest  InputSameDT=on
  1-D Lookup Table3 : Lookup_n-D  NumberOfTableDimensions=1  BreakpointsForDimension1=[0:3]  IndexSearchMethod=Evenly spaced points  Table=[-3 -3 3 -1]  InterpMethod=Flat  DiagnosticForOutOfRangeInput=Error  InternalRulePriority=Speed  OutDataTypeStr=fixdt(1,3,0)  RndMeth=Simplest  InputSameDT=on
  1-D Lookup Table4 : Lookup_n-D  NumberOfTableDimensions=1  BreakpointsForDimension1=[0:3]  IndexSearchMethod=Evenly spaced points  Table=[3 3 -3 -3]  InterpMethod=Flat  DiagnosticForOutOfRangeInput=Error  InternalRulePriority=Speed  OutDataTypeStr=fixdt(1,3,0)  RndMeth=Simplest  InputSameDT=on
  1-D Lookup Table5 : Lookup_n-D  NumberOfTableDimensions=1  BreakpointsForDimension1=[0:3]  IndexSearchMethod=Evenly spaced points  Table=[1 1 -3 -3]  InterpMethod=Flat  DiagnosticForOutOfRangeInput=Error  InternalRulePriority=Speed  OutDataTypeStr=fixdt(1,3,0)  RndMeth=Simplest  InputSameDT=on
  1-D Lookup Table6 : Lookup_n-D  NumberOfTableDimensions=1  BreakpointsForDimension1=[0:3]  IndexSearchMethod=Evenly spaced points  Table=[-1 -1 -3 -3]  InterpMethod=Flat  DiagnosticForOutOfRangeInput=Error  InternalRulePriority=Speed  OutDataTypeStr=fixdt(1,3,0)  RndMeth=Simplest  InputSameDT=on
  1-D Lookup Table7 : Lookup_n-D  NumberOfTableDimensions=1  BreakpointsForDimension1=[0:3]  IndexSearchMethod=Evenly spaced points  Table=[-3 -3 -3 -3]  InterpMethod=Flat  DiagnosticForOutOfRangeInput=Error  InternalRulePriority=Speed  OutDataTypeStr=fixdt(1,3,0)  RndMeth=Simplest  InputSameDT=on
  Out1 : Outport
  Out2 : Outport  Port=2
  Out3 : Outport  Port=3
  Out4 : Outport  Port=4
  Out5 : Outport  Port=5
  Out6 : Outport  Port=6
  Out7 : Outport  Port=7
  Out8 : Outport  Port=8
  wires:
  1-D Lookup Table7/1 -> Out8/1
  1-D Lookup Table2/1 -> Out3/1
  1-D Lookup Table/1 -> Out1/1
  1-D Lookup Table5/1 -> Out6/1
  1-D Lookup Table4/1 -> Out5/1
  1-D Lookup Table1/1 -> Out2/1
  1-D Lookup Table3/1 -> Out4/1
  enb/1 -> 1-D Lookup Table7/1, 1-D Lookup Table6/1, 1-D Lookup Table5/1, 1-D Lookup Table4/1, 1-D Lookup Table/1, 1-D Lookup Table1/1, 1-D Lookup Table2/1, 1-D Lookup Table3/1
  1-D Lookup Table6/1 -> Out7/1

== system lib_rfsoc_fec/Soft Demodulation/Soft Demodulation/Subsystem1 ==
  a : Inport
  b : Inport  Port=2
  a1 : Inport  Port=3
  b1 : Inport  Port=4
  a2 : Inport  Port=5
  b2 : Inport  Port=6
  a3 : Inport  Port=7
  b3 : Inport  Port=8
  get_min1 : Subsystem
  get_min2 : Subsystem
  get_min3 : Subsystem
  get_min4 : Subsystem
  get_min5 : Subsystem
  get_min6 : Subsystem
  get_min7 : Subsystem
  min : Outport
  wires:
  a2/1 -> get_min3/1(a)
  b/1 -> get_min1/2(b)
  a1/1 -> get_min2/1(a)
  b3/1 -> get_min4/2(b)
  get_min7/1(min) -> min/1
  get_min1/1(min) -> get_min5/1(a)
  a3/1 -> get_min4/1(a)
  get_min4/1(min) -> get_min6/2(b)
  get_min2/1(min) -> get_min5/2(b)
  b1/1 -> get_min2/2(b)
  get_min3/1(min) -> get_min6/1(a)
  get_min6/1(min) -> get_min7/2(b)
  a/1 -> get_min1/1(a)
  b2/1 -> get_min3/2(b)
  get_min5/1(min) -> get_min7/1(a)

== system lib_rfsoc_fec/Soft Demodulation/Soft Demodulation/Subsystem3 ==
  enb : Inport
  1-D Lookup Table : Lookup_n-D  NumberOfTableDimensions=1  BreakpointsForDimension1=[0:3]  IndexSearchMethod=Evenly spaced points  Table=[-3 1 3 3]  InterpMethod=Flat  DiagnosticForOutOfRangeInput=Error  InternalRulePriority=Speed  OutDataTypeStr=fixdt(1,3,0)  RndMeth=Simplest  InputSameDT=on
  1-D Lookup Table1 : Lookup_n-D  NumberOfTableDimensions=1  BreakpointsForDimension1=[0:3]  IndexSearchMethod=Evenly spaced points  Table=[-3 1 1 1]  InterpMethod=Flat  DiagnosticForOutOfRangeInput=Error  InternalRulePriority=Speed  OutDataTypeStr=fixdt(1,3,0)  RndMeth=Simplest  InputSameDT=on
  1-D Lookup Table2 : Lookup_n-D  NumberOfTableDimensions=1  BreakpointsForDimension1=[0:3]  IndexSearchMethod=Evenly spaced points  Table=[-3 1 -1 -1]  InterpMethod=Flat  DiagnosticForOutOfRangeInput=Error  InternalRulePriority=Speed  OutDataTypeStr=fixdt(1,3,0)  RndMeth=Simplest  InputSameDT=on
  1-D Lookup Table3 : Lookup_n-D  NumberOfTableDimensions=1  BreakpointsForDimension1=[0:3]  IndexSearchMethod=Evenly spaced points  Table=[-3 1 -3 -3]  InterpMethod=Flat  DiagnosticForOutOfRangeInput=Error  InternalRulePriority=Speed  OutDataTypeStr=fixdt(1,3,0)  RndMeth=Simplest  InputSameDT=on
  1-D Lookup Table4 : Lookup_n-D  NumberOfTableDimensions=1  BreakpointsForDimension1=[0:3]  IndexSearchMethod=Evenly spaced points  Table=[3 3 3 3]  InterpMethod=Flat  DiagnosticForOutOfRangeInput=Error  InternalRulePriority=Speed  OutDataTypeStr=fixdt(1,3,0)  RndMeth=Simplest  InputSameDT=on
  1-D Lookup Table5 : Lookup_n-D  NumberOfTableDimensions=1  BreakpointsForDimension1=[0:3]  IndexSearchMethod=Evenly spaced points  Table=[3 3 1 1]  InterpMethod=Flat  DiagnosticForOutOfRangeInput=Error  InternalRulePriority=Speed  OutDataTypeStr=fixdt(1,3,0)  RndMeth=Simplest  InputSameDT=on
  1-D Lookup Table6 : Lookup_n-D  NumberOfTableDimensions=1  BreakpointsForDimension1=[0:3]  IndexSearchMethod=Evenly spaced points  Table=[3 3 -1 -1]  InterpMethod=Flat  DiagnosticForOutOfRangeInput=Error  InternalRulePriority=Speed  OutDataTypeStr=fixdt(1,3,0)  RndMeth=Simplest  InputSameDT=on
  1-D Lookup Table7 : Lookup_n-D  NumberOfTableDimensions=1  BreakpointsForDimension1=[0:3]  IndexSearchMethod=Evenly spaced points  Table=[3 3 -3 -3]  InterpMethod=Flat  DiagnosticForOutOfRangeInput=Error  InternalRulePriority=Speed  OutDataTypeStr=fixdt(1,3,0)  RndMeth=Simplest  InputSameDT=on
  Out1 : Outport
  Out2 : Outport  Port=2
  Out3 : Outport  Port=3
  Out4 : Outport  Port=4
  Out5 : Outport  Port=5
  Out6 : Outport  Port=6
  Out7 : Outport  Port=7
  Out8 : Outport  Port=8
  wires:
  1-D Lookup Table7/1 -> Out8/1
  1-D Lookup Table2/1 -> Out3/1
  1-D Lookup Table/1 -> Out1/1
  1-D Lookup Table5/1 -> Out6/1
  1-D Lookup Table4/1 -> Out5/1
  1-D Lookup Table1/1 -> Out2/1
  1-D Lookup Table3/1 -> Out4/1
  enb/1 -> 1-D Lookup Table3/1, 1-D Lookup Table2/1, 1-D Lookup Table1/1, 1-D Lookup Table/1, 1-D Lookup Table7/1, 1-D Lookup Table6/1, 1-D Lookup Table5/1, 1-D Lookup Table4/1
  1-D Lookup Table6/1 -> Out7/1

== system lib_rfsoc_fec/Soft Demodulation/Soft Demodulation/Subsystem4 ==
  enb : Inport
  1-D Lookup Table : Lookup_n-D  NumberOfTableDimensions=1  BreakpointsForDimension1=[0:3]  IndexSearchMethod=Evenly spaced points  Table=[1 -3 3 3]  InterpMethod=Flat  DiagnosticForOutOfRangeInput=Error  InternalRulePriority=Speed  OutDataTypeStr=fixdt(1,3,0)  RndMeth=Simplest  InputSameDT=on
  1-D Lookup Table1 : Lookup_n-D  NumberOfTableDimensions=1  BreakpointsForDimension1=[0:3]  IndexSearchMethod=Evenly spaced points  Table=[1 -3 1 1]  InterpMethod=Flat  DiagnosticForOutOfRangeInput=Error  InternalRulePriority=Speed  OutDataTypeStr=fixdt(1,3,0)  RndMeth=Simplest  InputSameDT=on
  1-D Lookup Table2 : Lookup_n-D  NumberOfTableDimensions=1  BreakpointsForDimension1=[0:3]  IndexSearchMethod=Evenly spaced points  Table=[1 -3 -1 -1]  InterpMethod=Flat  DiagnosticForOutOfRangeInput=Error  InternalRulePriority=Speed  OutDataTypeStr=fixdt(1,3,0)  RndMeth=Simplest  InputSameDT=on
  1-D Lookup Table3 : Lookup_n-D  NumberOfTableDimensions=1  BreakpointsForDimension1=[0:3]  IndexSearchMethod=Evenly spaced points  Table=[1 -3 -3 -3]  InterpMethod=Flat  DiagnosticForOutOfRangeInput=Error  InternalRulePriority=Speed  OutDataTypeStr=fixdt(1,3,0)  RndMeth=Simplest  InputSameDT=on
  1-D Lookup Table4 : Lookup_n-D  NumberOfTableDimensions=1  BreakpointsForDimension1=[0:3]  IndexSearchMethod=Evenly spaced points  Table=[-1 -1 3 3]  InterpMethod=Flat  DiagnosticForOutOfRangeInput=Error  InternalRulePriority=Speed  OutDataTypeStr=fixdt(1,3,0)  RndMeth=Simplest  InputSameDT=on
  1-D Lookup Table5 : Lookup_n-D  NumberOfTableDimensions=1  BreakpointsForDimension1=[0:3]  IndexSearchMethod=Evenly spaced points  Table=[-1 -1 1 1]  InterpMethod=Flat  DiagnosticForOutOfRangeInput=Error  InternalRulePriority=Speed  OutDataTypeStr=fixdt(1,3,0)  RndMeth=Simplest  InputSameDT=on
  1-D Lookup Table6 : Lookup_n-D  NumberOfTableDimensions=1  BreakpointsForDimension1=[0:3]  IndexSearchMethod=Evenly spaced points  Table=[-1 -1 -1 -1]  InterpMethod=Flat  DiagnosticForOutOfRangeInput=Error  InternalRulePriority=Speed  OutDataTypeStr=fixdt(1,3,0)  RndMeth=Simplest  InputSameDT=on
  1-D Lookup Table7 : Lookup_n-D  NumberOfTableDimensions=1  BreakpointsForDimension1=[0:3]  IndexSearchMethod=Evenly spaced points  Table=[-1 -1 -3 -3]  InterpMethod=Flat  DiagnosticForOutOfRangeInput=Error  InternalRulePriority=Speed  OutDataTypeStr=fixdt(1,3,0)  RndMeth=Simplest  InputSameDT=on
  Out1 : Outport
  Out2 : Outport  Port=2
  Out3 : Outport  Port=3
  Out4 : Outport  Port=4
  Out5 : Outport  Port=5
  Out6 : Outport  Port=6
  Out7 : Outport  Port=7
  Out8 : Outport  Port=8
  wires:
  1-D Lookup Table6/1 -> Out7/1
  enb/1 -> 1-D Lookup Table/1, 1-D Lookup Table1/1, 1-D Lookup Table2/1, 1-D Lookup Table3/1, 1-D Lookup Table4/1, 1-D Lookup Table5/1, 1-D Lookup Table6/1, 1-D Lookup Table7/1
  1-D Lookup Table3/1 -> Out4/1
  1-D Lookup Table1/1 -> Out2/1
  1-D Lookup Table4/1 -> Out5/1
  1-D Lookup Table5/1 -> Out6/1
  1-D Lookup Table/1 -> Out1/1
  1-D Lookup Table2/1 -> Out3/1
  1-D Lookup Table7/1 -> Out8/1

== system lib_rfsoc_fec/Soft Demodulation/Soft Demodulation/Subsystem5 ==
  enb : Inport
  1-D Lookup Table : Lookup_n-D  NumberOfTableDimensions=1  BreakpointsForDimension1=[0:3]  IndexSearchMethod=Evenly spaced points  Table=[3 3 1 3]  InterpMethod=Flat  DiagnosticForOutOfRangeInput=Error  InternalRulePriority=Speed  OutDataTypeStr=fixdt(1,3,0)  RndMeth=Simplest  InputSameDT=on
  1-D Lookup Table1 : Lookup_n-D  NumberOfTableDimensions=1  BreakpointsForDimension1=[0:3]  IndexSearchMethod=Evenly spaced points  Table=[1 1 1 3]  InterpMethod=Flat  DiagnosticForOutOfRangeInput=Error  InternalRulePriority=Speed  OutDataTypeStr=fixdt(1,3,0)  RndMeth=Simplest  InputSameDT=on
  1-D Lookup Table2 : Lookup_n-D  NumberOfTableDimensions=1  BreakpointsForDimension1=[0:3]  IndexSearchMethod=Evenly spaced points  Table=[-1 -1 1 3]  InterpMethod=Flat  DiagnosticForOutOfRangeInput=Error  InternalRulePriority=Speed  OutDataTypeStr=fixdt(1,3,0)  RndMeth=Simplest  InputSameDT=on
  1-D Lookup Table3 : Lookup_n-D  NumberOfTableDimensions=1  BreakpointsForDimension1=[0:3]  IndexSearchMethod=Evenly spaced points  Table=[-3 -3 1 3]  InterpMethod=Flat  DiagnosticForOutOfRangeInput=Error  InternalRulePriority=Speed  OutDataTypeStr=fixdt(1,3,0)  RndMeth=Simplest  InputSameDT=on
  1-D Lookup Table4 : Lookup_n-D  NumberOfTableDimensions=1  BreakpointsForDimension1=[0:3]  IndexSearchMethod=Evenly spaced points  Table=[3 3 -1 1]  InterpMethod=Flat  DiagnosticForOutOfRangeInput=Error  InternalRulePriority=Speed  OutDataTypeStr=fixdt(1,3,0)  RndMeth=Simplest  InputSameDT=on
  1-D Lookup Table5 : Lookup_n-D  NumberOfTableDimensions=1  BreakpointsForDimension1=[0:3]  IndexSearchMethod=Evenly spaced points  Table=[1 1 -1 1]  InterpMethod=Flat  DiagnosticForOutOfRangeInput=Error  InternalRulePriority=Speed  OutDataTypeStr=fixdt(1,3,0)  RndMeth=Simplest  InputSameDT=on
  1-D Lookup Table6 : Lookup_n-D  NumberOfTableDimensions=1  BreakpointsForDimension1=[0:3]  IndexSearchMethod=Evenly spaced points  Table=[-1 -1 -1 1]  InterpMethod=Flat  DiagnosticForOutOfRangeInput=Error  InternalRulePriority=Speed  OutDataTypeStr=fixdt(1,3,0)  RndMeth=Simplest  InputSameDT=on
  1-D Lookup Table7 : Lookup_n-D  NumberOfTableDimensions=1  BreakpointsForDimension1=[0:3]  IndexSearchMethod=Evenly spaced points  Table=[-3 -3 -1 1]  InterpMethod=Flat  DiagnosticForOutOfRangeInput=Error  InternalRulePriority=Speed  OutDataTypeStr=fixdt(1,3,0)  RndMeth=Simplest  InputSameDT=on
  Out1 : Outport
  Out2 : Outport  Port=2
  Out3 : Outport  Port=3
  Out4 : Outport  Port=4
  Out5 : Outport  Port=5
  Out6 : Outport  Port=6
  Out7 : Outport  Port=7
  Out8 : Outport  Port=8
  wires:
  1-D Lookup Table7/1 -> Out8/1
  1-D Lookup Table2/1 -> Out3/1
  1-D Lookup Table/1 -> Out1/1
  1-D Lookup Table5/1 -> Out6/1
  1-D Lookup Table4/1 -> Out5/1
  1-D Lookup Table1/1 -> Out2/1
  1-D Lookup Table3/1 -> Out4/1
  enb/1 -> 1-D Lookup Table7/1, 1-D Lookup Table6/1, 1-D Lookup Table5/1, 1-D Lookup Table4/1, 1-D Lookup Table3/1, 1-D Lookup Table2/1, 1-D Lookup Table1/1, 1-D Lookup Table/1
  1-D Lookup Table6/1 -> Out7/1

== system lib_rfsoc_fec/Soft Demodulation/Soft Demodulation/Subsystem6 ==
  a : Inport
  b : Inport  Port=2
  a1 : Inport  Port=3
  b1 : Inport  Port=4
  a2 : Inport  Port=5
  b2 : Inport  Port=6
  a3 : Inport  Port=7
  b3 : Inport  Port=8
  get_min1 : Subsystem
  get_min2 : Subsystem
  get_min3 : Subsystem
  get_min4 : Subsystem
  get_min5 : Subsystem
  get_min6 : Subsystem
  get_min7 : Subsystem
  min : Outport
  wires:
  get_min5/1(min) -> get_min7/1(a)
  b2/1 -> get_min3/2(b)
  a/1 -> get_min1/1(a)
  get_min6/1(min) -> get_min7/2(b)
  get_min3/1(min) -> get_min6/1(a)
  b1/1 -> get_min2/2(b)
  get_min2/1(min) -> get_min5/2(b)
  get_min4/1(min) -> get_min6/2(b)
  a3/1 -> get_min4/1(a)
  get_min1/1(min) -> get_min5/1(a)
  get_min7/1(min) -> min/1
  b3/1 -> get_min4/2(b)
  a1/1 -> get_min2/1(a)
  b/1 -> get_min1/2(b)
  a2/1 -> get_min3/1(a)

== system lib_rfsoc_fec/QAM Mapping/Buffer/sample_and_hold/tvalid hold ==
  In1 : Inport
  Compare To Constant : simulink/Logic and Bit Operations/Compare To Constant  relop===  const=3  OutDataTypeStr=boolean
  HDL Counter : hdlsllib/Sources/HDL Counter  CountType=Count limited  CountInit=0  CountStep=1  CountMax=7  CountFromType=Initial value  CountFrom=0  CountResetPort=on  CountLoadPort=off  CountEnbPort=on  CountDirPort=off  CountDataType=Unsigned  CountWordLen=3  CountFracLen=0  CountSampTime=1
  OR : Logic  Operator=OR  IconShape=distinctive  AllPortsSameDT=off  OutDataTypeStr=boolean
  Sample and Hold1 : dspsigops/Sample and Hold  trig=Rising edge  initCond=0  latchinput=off
  " " : Outport
  wires:
  HDL Counter/1 -> Compare To Constant/1
  Compare To Constant/1 -> OR/1
  OR/1 -> Sample and Hold1/Trigger, HDL Counter/1
  Sample and Hold1/1 -> " "/1, HDL Counter/2
  In1/1 -> Sample and Hold1/1, OR/2

== system lib_rfsoc_fec/QAM Mapping/Buffer/sample_and_hold1/tvalid hold ==
  In1 : Inport
  Compare To Constant : simulink/Logic and Bit Operations/Compare To Constant  relop===  const=3  OutDataTypeStr=boolean
  HDL Counter : hdlsllib/Sources/HDL Counter  CountType=Count limited  CountInit=0  CountStep=1  CountMax=7  CountFromType=Initial value  CountFrom=0  CountResetPort=on  CountLoadPort=off  CountEnbPort=on  CountDirPort=off  CountDataType=Unsigned  CountWordLen=3  CountFracLen=0  CountSampTime=1
  OR : Logic  Operator=OR  IconShape=distinctive  AllPortsSameDT=off  OutDataTypeStr=boolean
  Sample and Hold1 : dspsigops/Sample and Hold  trig=Rising edge  initCond=0  latchinput=off
  " " : Outport
  wires:
  In1/1 -> OR/2, Sample and Hold1/1
  Sample and Hold1/1 -> HDL Counter/2, " "/1
  OR/1 -> HDL Counter/1, Sample and Hold1/Trigger
  Compare To Constant/1 -> OR/1
  HDL Counter/1 -> Compare To Constant/1

== system lib_rfsoc_fec/QAM Mapping/Buffer/sample_and_hold2/tvalid hold ==
  In1 : Inport
  Compare To Constant : simulink/Logic and Bit Operations/Compare To Constant  relop===  const=3  OutDataTypeStr=boolean
  HDL Counter : hdlsllib/Sources/HDL Counter  CountType=Count limited  CountInit=0  CountStep=1  CountMax=7  CountFromType=Initial value  CountFrom=0  CountResetPort=on  CountLoadPort=off  CountEnbPort=on  CountDirPort=off  CountDataType=Unsigned  CountWordLen=3  CountFracLen=0  CountSampTime=1
  OR : Logic  Operator=OR  IconShape=distinctive  AllPortsSameDT=off  OutDataTypeStr=boolean
  Sample and Hold1 : dspsigops/Sample and Hold  trig=Rising edge  initCond=0  latchinput=off
  " " : Outport
  wires:
  HDL Counter/1 -> Compare To Constant/1
  Compare To Constant/1 -> OR/1
  OR/1 -> Sample and Hold1/Trigger, HDL Counter/1
  Sample and Hold1/1 -> " "/1, HDL Counter/2
  In1/1 -> Sample and Hold1/1, OR/2

== system lib_rfsoc_fec/QAM Mapping/Buffer/sample_and_hold3/tvalid hold ==
  In1 : Inport
  Compare To Constant : simulink/Logic and Bit Operations/Compare To Constant  relop===  const=3  OutDataTypeStr=boolean
  HDL Counter : hdlsllib/Sources/HDL Counter  CountType=Count limited  CountInit=0  CountStep=1  CountMax=7  CountFromType=Initial value  CountFrom=0  CountResetPort=on  CountLoadPort=off  CountEnbPort=on  CountDirPort=off  CountDataType=Unsigned  CountWordLen=3  CountFracLen=0  CountSampTime=1
  OR : Logic  Operator=OR  IconShape=distinctive  AllPortsSameDT=off  OutDataTypeStr=boolean
  Sample and Hold1 : dspsigops/Sample and Hold  trig=Rising edge  initCond=0  latchinput=off
  " " : Outport
  wires:
  In1/1 -> OR/2, Sample and Hold1/1
  Sample and Hold1/1 -> HDL Counter/2, " "/1
  OR/1 -> HDL Counter/1, Sample and Hold1/Trigger
  Compare To Constant/1 -> OR/1
  HDL Counter/1 -> Compare To Constant/1

== system lib_rfsoc_fec/QAM Mapping/QAM Mapping/N-Width QAM-16 Symbol Mapping Imag/QAM-16 Symbol Mapping 0 ==
  bits : Inport
  Bit Slice1 : hdlsllib/Logic and Bit Operations/Bit Slice  lidx=n+1  ridx=n
      settings: SourceProductBaseCode=SL
  Constant1 : Constant  Value=3  OutDataTypeStr=fixdt(1,3,0)  SampleTime=-1
  Constant2 : Constant  OutDataTypeStr=fixdt(1,3,0)  SampleTime=-1
  Constant3 : Constant  Value=-1  OutDataTypeStr=fixdt(1,3,0)  SampleTime=-1
  Constant4 : Constant  Value=-3  OutDataTypeStr=fixdt(1,3,0)  SampleTime=-1
  Multiport Switch1 : MultiPortSwitch  DataPortOrder=Zero-based contiguous  Inputs=4  zeroidx=on
  Q : Outport
  wires:
  Constant2/1 -> Multiport Switch1/3
  Constant1/1 -> Multiport Switch1/2
  Constant4/1 -> Multiport Switch1/4
  Constant3/1 -> Multiport Switch1/5
  bits/1 -> Bit Slice1/1
  Multiport Switch1/1 -> Q/1
  Bit Slice1/1 -> Multiport Switch1/1
